simulink model "Subsystem"  (R2020a)
settings: Solver=ode45  StartTime=0.0  StopTime=40  MaxStep=0.01  RelTol=1e-3
model workspace (MAT data in the model file):
  Ki = Simulink.Parameter
  Ki.Value = 32
  Ki.DataType = 'auto'
  Ki.Dimensions = [1 1]
  Kp = Simulink.Parameter
  Kp.Value = 274
  Kp.DataType = 'auto'
  Kp.Dimensions = [1 1]
  Ts = Simulink.Parameter
  Ts.Value = 0
  Ts.DataType = 'auto'
  Ts.Dimensions = [1 1]
settings Model: Creator=DELL  LastModifiedBy=DELL
settings DataIOCC: SaveOutput=off  SaveTime=off
settings DebuggingCC: ModelReferenceExtraNoncontSigs=none

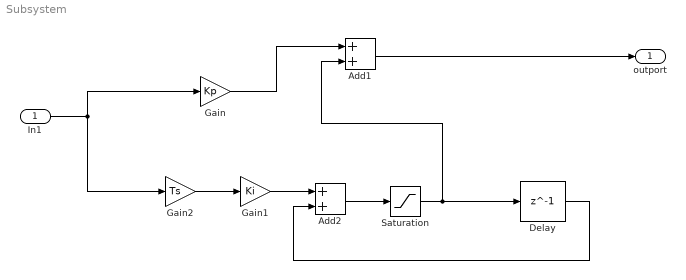
== system Subsystem ==
  In1 : Inport  OutDataTypeStr=double  PortDimensions=1  SampleTime=0
  Add1 : Sum
  Add2 : Sum
  Delay : Delay  DelayLength=1
  Gain : Gain  Gain=Kp
  Gain1 : Gain  Gain=Ki
  Gain2 : Gain  Gain=Ts
  Saturation : Saturate
  outport : Outport  OutDataTypeStr=double  PortDimensions=1  SampleTime=0
  wires:
  Gain2/1 -> Gain1/1
  Add2/1 -> Saturation/1
  Add1/1 -> outport/1
  In1/1 -> Gain2/1, Gain/1
  Gain/1 -> Add1/1
  Delay/1 -> Add2/2
  Saturation/1 -> Delay/1, Add1/2
  Gain1/1 -> Add2/1
